simulink model "ABS_System"  (R2021b)
settings: Solver=FixedStepAuto  StartTime=0.0  StopTime=25  FixedStep=0.01  RelTol=1e-3
values from neighbouring files (symbols this model uses):
  g = 9.81    [ABSData.m]
  I = 5    [ABSData.m]
  m = 75    [ABSData.m]
  R = 1.25    [ABSData.m]
  v0 = 44    [ABSData.m]
settings Model: Creator=14219  LastModifiedBy=14219

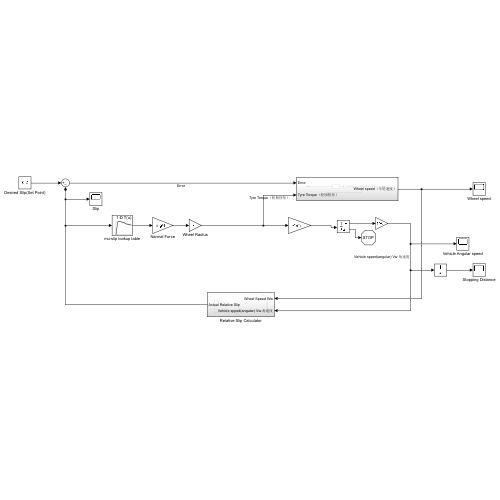
[thumbnail: Simulink's stored preview of the top-level diagram]
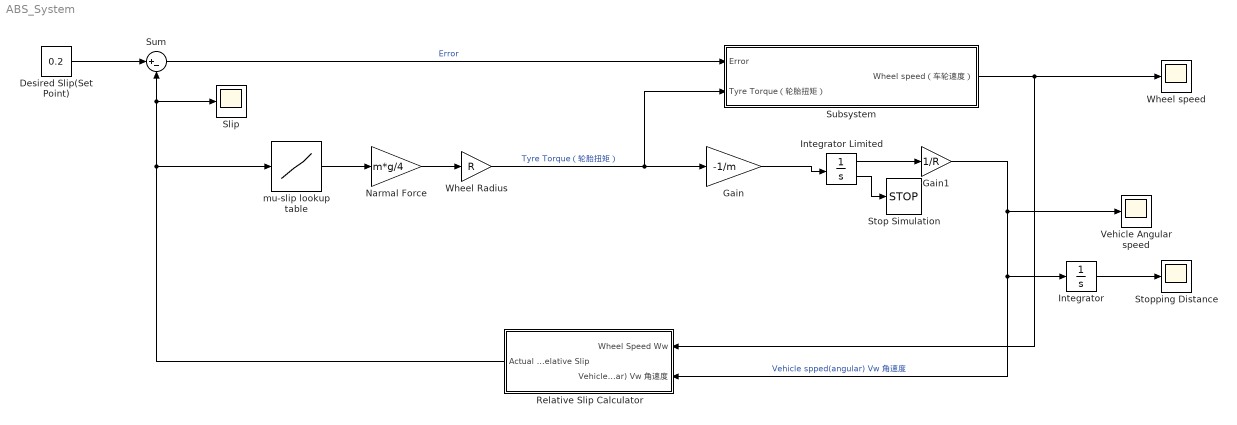
== system ABS_System ==
  Desired Slip(Set Point) : Constant  Value=0.2
  Gain : Gain  Gain=-1/m
  Gain1 : Gain  Gain=1/R
  Integrator : Integrator
  Integrator Limited : Integrator  InitialCondition=v0  LimitOutput=on  UpperSaturationLimit=1000  LowerSaturationLimit=0  ShowSaturationPort=on
  Narmal Force : Gain  Gain=m*g/4
  Relative Slip Calculator : Subsystem
  Slip : Scope
  Stop Simulation : Stop
  Stopping Distance : Scope
  Subsystem : Subsystem
  Sum : Sum  Inputs=|+-
  Vehicle Angular speed : Scope
  Wheel Radius : Gain  Gain=R
  Wheel speed : Scope
  mu-slip lookup table : Lookup_n-D  NumberOfTableDimensions=1  BreakpointsForDimension1=[0,0.05,0.1,0.15,0.2,0.25,0.3,0.35,0.4,0.45,0.5,0.55,0.6,0.65,0.7,0.75,0.8,0.85,0.9,0.95,1]  Table=[0,0.4,0.8,0.97,1,0.98,0.96,0.94,0.92,0.9,0.88,0.855,0.83,0.81,0.79,0.77,0.75,0.73,0.72,0.71,0.7]  InternalRulePriority=Speed  RndMeth=Simplest  InputSameDT=on
  wires:
  Desired Slip(Set Point)/1 -> Sum/1
  mu-slip lookup table/1 -> Narmal Force/1
  Narmal Force/1 -> Wheel Radius/1
  Sum/1 -> Subsystem/1(Error)  "Error"
  Wheel Radius/1 -> Gain/1, Subsystem/2(Tyre Torque（轮胎扭矩）)  "Tyre Torque（轮胎扭矩）"
  Subsystem/1(Wheel speed（车轮速度）) -> Wheel speed/1, Relative Slip Calculator/1(Wheel Speed Ww)
  Gain/1 -> Integrator Limited/1
  Integrator Limited/1 -> Gain1/1
  Gain1/1 -> Relative Slip Calculator/2(Vehicle spped(angular) Vw 角速度), Integrator/1, Vehicle Angular speed/1  "Vehicle spped(angular) Vw 角速度"
  Integrator Limited/2 -> Stop Simulation/1
  Integrator/1 -> Stopping Distance/1
  Relative Slip Calculator/1(Actual Relative Slip) -> mu-slip lookup table/1, Slip/1, Sum/2

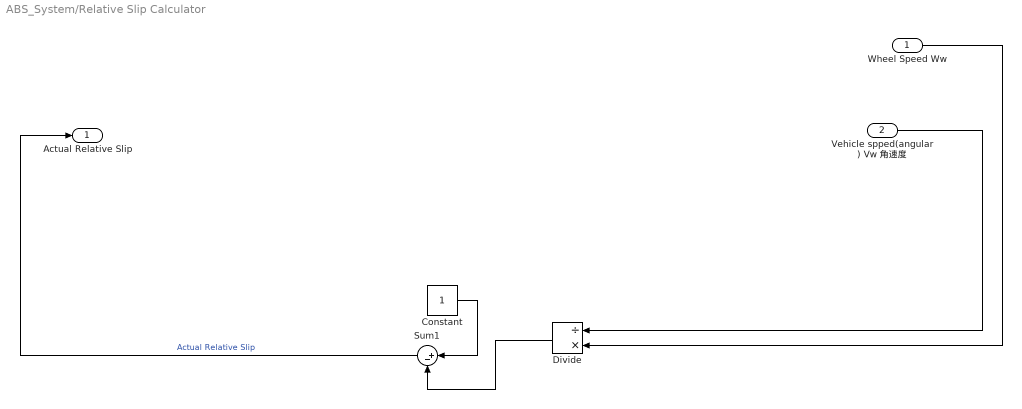
== system ABS_System/Relative Slip Calculator ==
  Wheel Speed Ww : Inport
  Vehicle spped(angular) Vw 角速度 : Inport  Port=2
  Constant : Constant
  Divide : Product  Inputs=/*
  Sum1 : Sum  Inputs=|+-
  Actual Relative Slip : Outport
  wires:
  Wheel Speed Ww/1 -> Divide/2
  Sum1/1 -> Actual Relative Slip/1  "Actual Relative Slip"
  Constant/1 -> Sum1/1
  Divide/1 -> Sum1/2
  Vehicle spped(angular) Vw 角速度/1 -> Divide/1

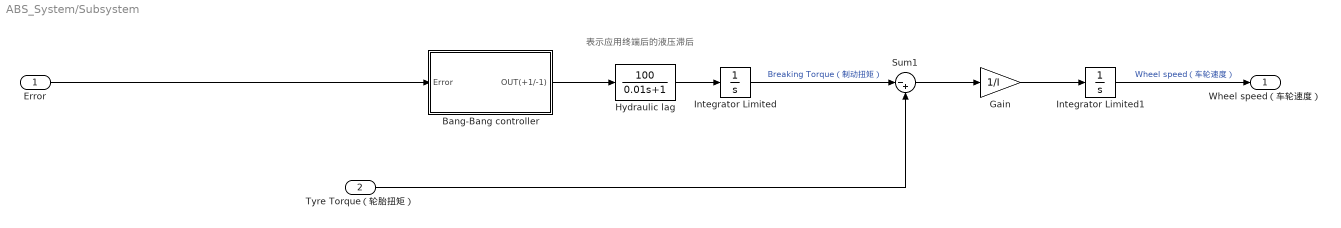
== system ABS_System/Subsystem ==
  note: 表示应用终端后的液压滞后
  Error : Inport
  Tyre Torque（轮胎扭矩） : Inport  Port=2
  Bang-Bang controller : Subsystem
  Gain : Gain  Gain=1/I
  Hydraulic lag : TransferFcn  Numerator=[100]  Denominator=[0.01 1]
  Integrator Limited : Integrator  LimitOutput=on  UpperSaturationLimit=1000  LowerSaturationLimit=0
  Integrator Limited1 : Integrator  InitialCondition=v0/R  LimitOutput=on  UpperSaturationLimit=1000  LowerSaturationLimit=0
  Sum1 : Sum  Inputs=|-+
  Wheel speed（车轮速度） : Outport
  wires:
  Integrator Limited1/1 -> Wheel speed（车轮速度）/1  "Wheel speed（车轮速度）"
  Hydraulic lag/1 -> Integrator Limited/1
  Bang-Bang controller/1(OUT(+1/-1)) -> Hydraulic lag/1
  Gain/1 -> Integrator Limited1/1
  Integrator Limited/1 -> Sum1/1  "Breaking Torque（制动扭矩）"
  Error/1 -> Bang-Bang controller/1(Error)
  Sum1/1 -> Gain/1
  Tyre Torque（轮胎扭矩）/1 -> Sum1/2

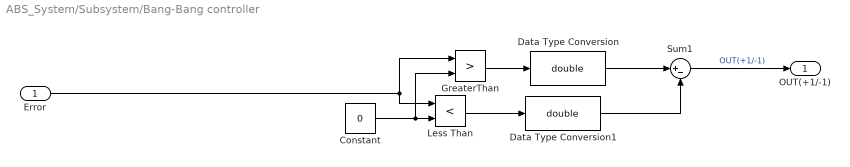
== system ABS_System/Subsystem/Bang-Bang controller ==
  Error : Inport
  Constant : Constant  Value=0
  Data Type Conversion : DataTypeConversion  OutDataTypeStr=double  RndMeth=Zero
  Data Type Conversion1 : DataTypeConversion  OutDataTypeStr=double  RndMeth=Zero
  GreaterThan : RelationalOperator  Operator=>  OutDataTypeStr=boolean  RndMeth=Simplest
  Less Than : RelationalOperator  Operator=<  OutDataTypeStr=boolean  RndMeth=Simplest
  Sum1 : Sum  Inputs=|+-
  OUT(+1/-1) : Outport
  wires:
  Data Type Conversion/1 -> Sum1/1
  GreaterThan/1 -> Data Type Conversion/1
  Constant/1 -> GreaterThan/2, Less Than/2
  Data Type Conversion1/1 -> Sum1/2
  Less Than/1 -> Data Type Conversion1/1
  Error/1 -> GreaterThan/1, Less Than/1
  Sum1/1 -> OUT(+1/-1)/1  "OUT(+1/-1)"
